simulink model "DTC"  (R2023a)
settings: Solver=FixedStepAuto  StartTime=0.0  StopTime=6  FixedStep=Ts  MaxStep=1e-4  RelTol=1e-3
PreLoadFcn:
  | Ts=1e-5;
InitFcn:
  | Ts=1e-5;
undefined symbols (not defined in the file): DiscIntNeverNeededParam
libraries: spsIGBTDiodeLib x6, slpidlib x2, spsAsynchronousMachineSIUnitsLib x1, simulink x1, spsDCVoltageSourceLib x1, spsVoltageMeasurementLib x1, sps_lib x1
Description:
  | Copyright 2011-2013 Ruan Jiayang, Tsinghua Univ.
settings Model: ExtModeTrigMode=oneshot  Creator=Hoang Lehuy, Laval University  LastModifiedBy=搬砖工卢卡斯
settings SolverCC: AlgebraicLoopSolver=TrustRegion
settings DataIOCC: SaveFinalState=on  SaveFormat=Array  SignalLoggingSaveFormat=ModelDataLogs  SaveOutput=off  SaveTime=off  ReturnWorkspaceOutputs=off  SignalLoggingName=sigsOut
settings OptimizationCC: BlockReduction=off  ExpressionDepthLimit=2147483647  InitFltsAndDblsToZero=on  LifeSpan=inf
settings DebuggingCC: SaveWithParameterizedLinksMsg=none  UnderspecifiedInitializationDetection=Classic  MergeDetectMultiDrivingBlocksExec=none  CheckExecutionContextPreStartOutputMsg=on  SignalResolutionControl=TryResolveAllWithWarning  MultiTaskDSMMsg=warning  MultiTaskCondExecSysMsg=none  FcnCallInpInsideContextMsg=warning  UnconnectedInputMsg=warning  UnconnectedLineMsg=warning  StateNameClashWarn=warning  SFUnexpectedBacktrackingDiag=warning  SFNoUnconditionalDefaultTransitionDiag=warning  SFExecutionAtInitializationDiag=none  ArithmeticOperatorsInVariantConditions=warning
settings HardwareCC: ProdBitPerPointer=32  ProdBitPerSizeT=32  ProdBitPerPtrDiffT=32  ProdLargestAtomicFloat=None  ProdIntDivRoundTo=Undefined  ProdEndianess=Unspecified  ProdWordSize=32  ProdHWDeviceType=32-bit Generic  TargetUnknown=on
settings ModelReferenceCC: PropagateSignalLabelsOutOfModel=off
settings SFSimCC: SimUseLocalCustomCode=off  SimParseCustomCode=off  CustomCodeUndefinedFunction=UseInterfaceOnly
settings RTWCC: RTWUseLocalCustomCode=off
settings CodeAppCC: StateflowObjectComments=on
settings GRTTargetCC: TargetFcnLib=ansi_tfl_tmw.mat  TargetLangStandard=C89/C90 (ANSI)  CombineOutputUpdateFcns=off  GRTInterface=on
settings ConfigComp: CovMetricSettings=dw  CovSaveCumulativeToWorkspaceVar=on  CovSaveSingleToWorkspaceVar=on  CovExternalEMLEnable=off

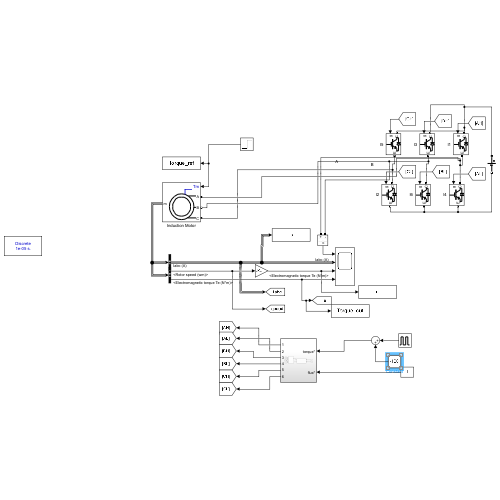
[thumbnail: Simulink's stored preview of the top-level diagram]
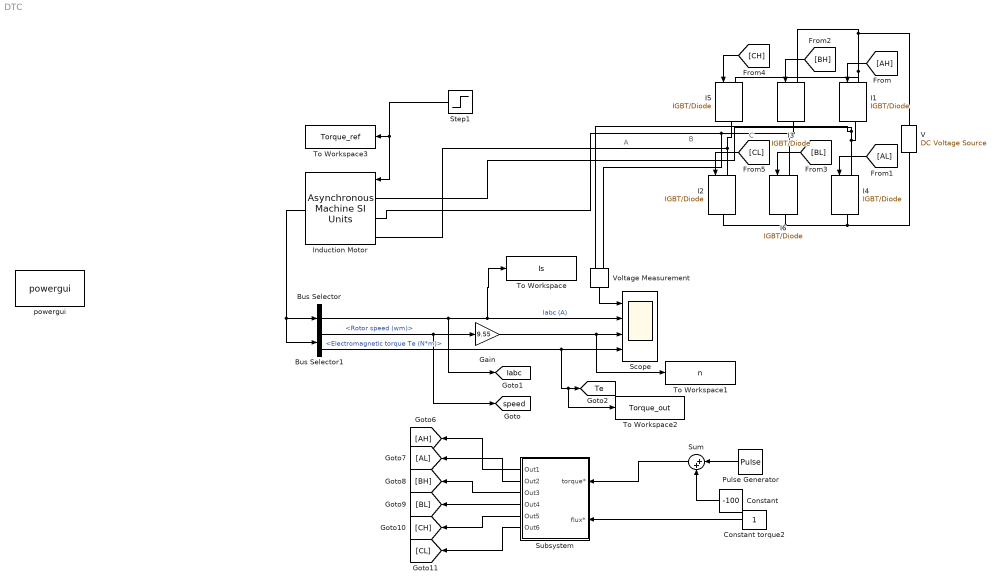
== system DTC ==
  note: B
  note: A
  note: C
  Bus Selector : BusSelector  OutputSignals=Stator measurements.Stator current is_a (A),Stator measurements.Stator current is_b (A),Stator measurements.Stator current is_c (A)  OutputAsBus=on
  Bus Selector1 : BusSelector  OutputSignals=Mechanical.Rotor speed (wm),Mechanical.Electromagnetic torque Te (N*m)
  Constant : Constant  Value=-100
  Constant torque2 : Constant
  Gain : Gain  Gain=9.55
  I{1..6} (6 alike) : spsIGBTDiodeLib/IGBT//Diode  Ron=1e-3  Rs=1e5  Cs=inf  Measurements=off
  "Induction Motor " : spsAsynchronousMachineSIUnitsLib/Asynchronous Machine SI Units  RotorType=Squirrel-cage  PresetModel=No  MechanicalLoad=Torque Tm  ShowDetailedParameters=on  ReferenceFrame=Stationary  Units=SI  MeasurementBus=off  NominalParameters=[ 2000, 346, 60 ]  VoltageRatio=1  Stator=[ 0.087 0.8e-3 ]  Rotor="[ 0.228  0.8e-3 ]"  Cage1=[0.4155 0.002066]  Cage2=[0.4168 0.0003495]  Lm=34.7e-3  Mechanical="[1.662  0.01 2 ]"  PolePairs=2  InitialConditions="[ 1, 0 ,  0 , 0 , 0 , 0 , 0 , 0 ]"  SimulateSaturation=off  Saturation=[0 0;0 0]  LoadFlowParameters=0  TsPowergui=0  TsBlock=-1  IterativeModel=Trapezoidal non iterative  IterativeDiscreteModel=Trapezoidal non iterative  Pmec=1.492e+006
      settings: AttributesFormatString=\n
  Pulse Generator : DiscretePulseGenerator  PulseType=Time based  Amplitude=200  PulseWidth=50
  Scope : Scope  NumInputPorts=4
  Step1 : Step  Time=1.5  After=0  SampleTime=0
  Subsystem : Subsystem
  Sum : Sum  Inputs=|++
  To Workspace : ToWorkspace  VariableName=Is  SaveFormat=Timeseries  SampleTime=-1
  To Workspace1 : ToWorkspace  VariableName=n  SaveFormat=Timeseries  SampleTime=-1
  To Workspace2 : ToWorkspace  VariableName=Torque_out  SaveFormat=Timeseries  SampleTime=-1
  To Workspace3 : ToWorkspace  VariableName=Torque_ref  SaveFormat=Timeseries  SampleTime=-1
  V : spsDCVoltageSourceLib/DC Voltage Source  Amplitude=530  Measurements=None
  Voltage Measurement : spsVoltageMeasurementLib/Voltage Measurement  PhasorSimulation=off  OutputType=Complex  PSBequivalent=0
  powergui : sps_lib/powergui  Priority=2  SimulationMode=Discrete  SampleTime=Ts  frequency=60  Iterations=50  frequencyindice=0  Pbase=100e6  ErrMax=1e-4  UnitsV=kV  UnitsW=MW  buscounter=0  FunctionMessages=off  echomessages=off  EnableUseOfTLC=off  CurrentSourceSwitches=on  DisableSnubberDevices=off  DisableRonSwitches=off  DisableVfSwitches=off  DisplayEquations=off  AutomaticDiscreteSolvers=off  SolverType=Tustin/Backward Euler (TBE)  Interpol=off  ExternalGateDelay=off  methode=off  Ts=0  x0status=blocks  SPID=off  SwTol=0  HookPort=off  NonlinearTolerance=1e-4  nMaxIteration=100  ContinueOnMaxIteration=off  RestoreLinks=warning  ResistiveCurrentMeasurement=off  Frange=[0:2:500]  Ylog=off  Xlog=on  ShowGrid=off  save=off  variable=ZData  structure=0  ZoomFFT=on  StartTime=0.0  cycles=1  DisplayStyle=off  fundamental=60  FreqAxis=off  MaxFrequency=1000  frequencyindicesteady=1  RmsSteady=1  display=off
  tag scope: Iabc=global, Te=global, speed=global
  wires:
  Bus Selector1/1 -> Gain/1, [speed]  "<Rotor speed (wm)>"
  Bus Selector/1 -> [Iabc], To Workspace/1, Scope/2  "Iabc (A)"
  Bus Selector1/2 -> Scope/4, To Workspace2/1, [Te]  "<Electromagnetic torque Te (N*m)>"
  "Induction Motor "/1 -> Bus Selector1/1, Bus Selector/1
  Gain/1 -> To Workspace1/1, Scope/3
  Constant torque2/1 -> Subsystem/2(flux*)
  Step1/1 -> "Induction Motor "/1, To Workspace3/1
  Voltage Measurement/1 -> Scope/1
  [CH] -> I5/1
  [BL] -> I6/1
  [BH] -> I3/1
  [AL] -> I4/1
  [CL] -> I2/1
  [AH] -> I1/1
  Subsystem/1(Out1) -> [AH]
  Subsystem/2(Out2) -> [AL]
  Subsystem/3(Out3) -> [BH]
  Subsystem/4(Out4) -> [BL]
  Subsystem/5(Out5) -> [CH]
  Subsystem/6(Out6) -> [CL]
  Pulse Generator/1 -> Sum/1
  Constant/1 -> Sum/2
  Sum/1 -> Subsystem/1(torque*)
  connections:
  Voltage Measurement/LConn2 -- I6/LConn1 -- I3/RConn1 -- "Induction Motor "/LConn2
  I3/LConn1 -- V/RConn1 -- I5/LConn1 -- I1/LConn1
  I4/RConn1 -- V/LConn1 -- I2/RConn1 -- I6/RConn1
  Voltage Measurement/LConn1 -- "Induction Motor "/LConn1 -- I1/RConn1 -- I4/LConn1
  I5/RConn1 -- "Induction Motor "/LConn3 -- I2/LConn1

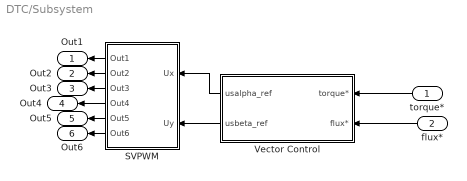
== system DTC/Subsystem ==
  torque* : Inport
  flux* : Inport  Port=2
  SVPWM : Subsystem
  Vector Control : Subsystem
  Out1 : Outport
  Out2 : Outport  Port=2
  Out3 : Outport  Port=3
  Out4 : Outport  Port=4
  Out5 : Outport  Port=5
  Out6 : Outport  Port=6
  wires:
  SVPWM/1(Out1) -> Out1/1
  SVPWM/5(Out5) -> Out5/1
  SVPWM/6(Out6) -> Out6/1
  flux*/1 -> Vector Control/2(flux*)
  Vector Control/2(usbeta_ref) -> SVPWM/2(Uy)
  Vector Control/1(usalpha_ref) -> SVPWM/1(Ux)
  torque*/1 -> Vector Control/1(torque*)
  SVPWM/2(Out2) -> Out2/1
  SVPWM/4(Out4) -> Out4/1
  SVPWM/3(Out3) -> Out3/1

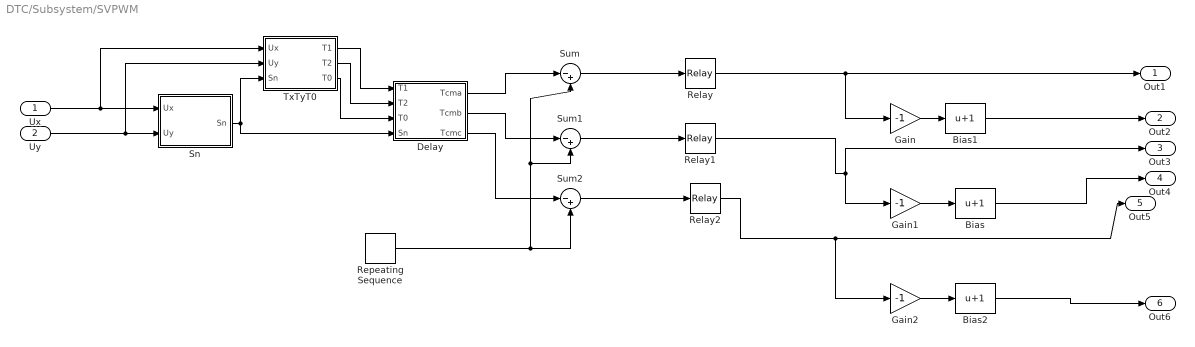
== system DTC/Subsystem/SVPWM ==
  Ux : Inport
  Uy : Inport  Port=2
  Bias : Bias  Bias=1  SaturateOnIntegerOverflow=off
  Bias1 : Bias  Bias=1  SaturateOnIntegerOverflow=off
  Bias2 : Bias  Bias=1  SaturateOnIntegerOverflow=off
  Delay : MATLAB Function  TreatAsAtomicUnit=on
  Gain : Gain  Gain=-1
  Gain1 : Gain  Gain=-1
  Gain2 : Gain  Gain=-1
  Relay : Relay  OnSwitchValue=0  OffSwitchValue=0
  Relay1 : Relay  OnSwitchValue=0  OffSwitchValue=0
  Relay2 : Relay  OnSwitchValue=0  OffSwitchValue=0
  Repeating Sequence : simulink/Sources/Repeating Sequence  rep_seq_t=[0 1/2000/2 1/2000]  rep_seq_y=[0 1/2000/2 0]
  Sn : MATLAB Function  TreatAsAtomicUnit=on
  Sum : Sum  Inputs=|-+
  Sum1 : Sum  Inputs=|-+
  Sum2 : Sum  Inputs=|-+
  TxTyT0 : MATLAB Function  TreatAsAtomicUnit=on
  Out1 : Outport
  Out2 : Outport  Port=2
  Out3 : Outport  Port=3
  Out4 : Outport  Port=4
  Out5 : Outport  Port=5
  Out6 : Outport  Port=6
  wires:
  Delay/1(Tcma) -> Sum/1
  Delay/2(Tcmb) -> Sum1/1
  Delay/3(Tcmc) -> Sum2/1
  Repeating Sequence/1 -> Sum/2, Sum1/2, Sum2/2
  Sum/1 -> Relay/1
  Sum2/1 -> Relay2/1
  Sum1/1 -> Relay1/1
  Relay1/1 -> Out3/1, Gain1/1
  Relay2/1 -> Out5/1, Gain2/1
  Sn/1(Sn) -> TxTyT0/3(Sn), Delay/4(Sn)
  TxTyT0/1(T1) -> Delay/1(T1)
  TxTyT0/2(T2) -> Delay/2(T2)
  TxTyT0/3(T0) -> Delay/3(T0)
  Gain1/1 -> Bias/1
  Gain/1 -> Bias1/1
  Gain2/1 -> Bias2/1
  Bias1/1 -> Out2/1
  Bias/1 -> Out4/1
  Bias2/1 -> Out6/1
  Relay/1 -> Out1/1, Gain/1
  Ux/1 -> Sn/1(Ux), TxTyT0/1(Ux)
  Uy/1 -> Sn/2(Uy), TxTyT0/2(Uy)

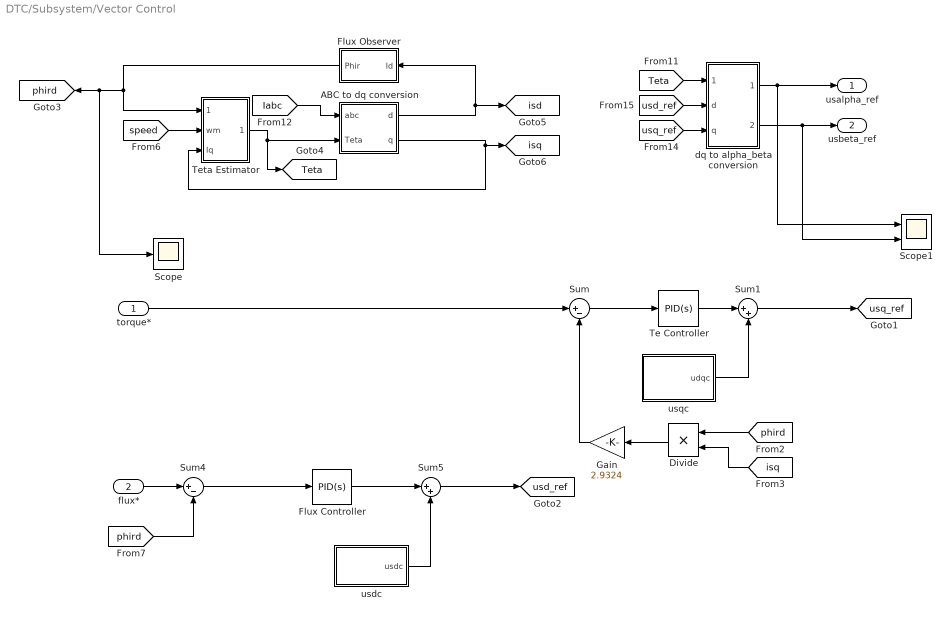
== system DTC/Subsystem/Vector Control ==
  torque* : Inport
  flux* : Inport  Port=2
  ABC to dq conversion : Subsystem
  Divide : Product
  Flux Controller : slpidlib/PID Controller  Controller=PID  Form=Parallel  TimeDomain=Continuous-time  UseExternalTs=off  SampleTime=1  IntegratorMethod=Forward Euler  FilterMethod=Forward Euler  ControllerParametersSource=internal  P=138.2107  I=247.3835  UseKiTs=off  D=0  N=100  UseFilter=on  TunerSelectOption=Transfer Function Based (PID Tuner App)  InitialConditionSource=internal  InitialConditionForIntegrator=100  InitialConditionForFilter=0  DifferentiatorICPrevScaledInput=0  ExternalReset=none  TrackingMode=off  Kt=1  LimitOutput=on  SatLimitsSource=internal  UpperSaturationLimit=200  LowerSaturationLimit=-200  LinearizeAsGain=off  AntiWindupMode=clamping  Kb=1  LimitIntegrator=off  UpperIntegratorSaturationLimit=inf  LowerIntegratorSaturationLimit=-inf  POutMin=[]  POutMax=[]  IOutMin=[]  IOutMax=[]  DOutMin=[]  DOutMax=[]  NOutMin=[]  NOutMax=[]  SumOutMin=[]  SumOutMax=[]  SaturationOutMin=[]  SaturationOutMax=[]  PParamMin=[]  PParamMax=[]  IParamMin=[]  IParamMax=[]  DParamMin=[]  DParamMax=[]  NParamMin=[]  NParamMax=[]  KbParamMin=[]  KbParamMax=[]  KtParamMin=[]  KtParamMax=[]  KbOutMin=[]  KbOutMax=[]  KtOutMin=[]  KtOutMax=[]  IntegratorOutMin=[]  IntegratorOutMax=[]  FilterOutMin=[]  FilterOutMax=[]  SumI1OutMin=[]  SumI1OutMax=[]  SumI2OutMin=[]  SumI2OutMax=[]  SumI3OutMin=[]  SumI3OutMax=[]  SumI4OutMin=[]  SumI4OutMax=[]  SumDOutMin=[]  SumDOutMax=[]  DifferentiatorOutMin=[]  DifferentiatorOutMax=[]  FilterDiffOutCoefMin=[]  FilterDiffOutCoefMax=[]  ReciprocalOutMin=[]  ReciprocalOutMax=[]  SumDenOutMin=[]  SumDenOutMax=[]  SumNumOutMin=[]  SumNumOutMax=[]  DivideOutMin=[]  DivideOutMax=[]  UdiffTsProdOutMin=[]  UdiffTsProdOutMax=[]  NTsProdOutMin=[]  NTsProdOutMax=[]  UintegralTsProdOutMin=[]  UintegralTsProdOutMax=[]  UngainTsProdOutMin=[]  UngainTsProdOutMax=[]  ClampingZeroOutDataTypeStr=Inherit: Inherit via back propagation  ClampingZeroOutMin=[]  ClampingZeroOutMax=[]  FilterDenConstantOutDataTypeStr=Inherit: Inherit via back propagation  FilterDenConstantOutMin=[]  FilterDenConstantOutMax=[]  PCopyOutDataTypeStr=Inherit: Inherit via back propagation  PCopyOutMin=[]  PCopyOutMax=[]  NCopyOutDataTypeStr=Inherit: Inherit via back propagation  NCopyOutMin=[]  NCopyOutMax=[]  IntegratorContinuousStateAttributes=''  IntegratorStateMustResolveToSignalObject=off  IntegratorRTWStateStorageClass=Auto  FilterContinuousStateAttributes=''  FilterStateMustResolveToSignalObject=off  FilterRTWStateStorageClass=Auto  ParallelPVariant=InternalParameters  IdealPVariant=Disabled  IVariant=InternalParameters  DVariant=InternalParameters  IntegratorVariant=Continuous  SatVariant=Enabled  AWVariant=ContClampingParallel  PCopyVariant=Disabled  TRVariant=Disabled  FdbkBlocksVariant=Forward  IdealPFdbkVariant=Disabled  SatFdbkVariant=Disabled  DerivativeFilterVariant=ContFilter  NVariant=InternalParameters  NCopyVariant=Disabled  FilterICVariant=InternalICsFilter  IntegratorICVariant=InternalICs  ExternalResetVariant=Disabled  TRSumVariant=Passthrough  SumFdbkVariant=Disabled  SumVariant=Sum_PID  TsampFilterVariant=InternalTs  TsampNgainVariant=Passthrough  TsampIntegralVariant=Disabled_SignalSpec  ExternalSaturationOutDataTypeStr=Inherit: Same as second input
  Flux Observer : Subsystem  mask(Flux Calcultation){}
      mask init:
      | NF=0.44572610323020e-6;
      | DF=[1 -0.99998715486734];
  Gain : Gain  Gain=2.9324
  Scope : Scope
  Scope1 : Scope  NumInputPorts=2
  Sum : Sum  Inputs=|+-
  Sum1 : Sum  Inputs=|++
  Sum4 : Sum  Inputs=|+-
  Sum5 : Sum  Inputs=|++
  Te Controller : slpidlib/PID Controller  Controller=PID  Form=Parallel  TimeDomain=Continuous-time  UseExternalTs=off  SampleTime=1  IntegratorMethod=Forward Euler  FilterMethod=Forward Euler  ControllerParametersSource=internal  P=2.69732  I=148.34534  UseKiTs=off  D=0  N=100  UseFilter=on  TunerSelectOption=Transfer Function Based (PID Tuner App)  InitialConditionSource=internal  InitialConditionForIntegrator=100  InitialConditionForFilter=0  DifferentiatorICPrevScaledInput=0  ExternalReset=none  TrackingMode=off  Kt=1  LimitOutput=on  SatLimitsSource=internal  UpperSaturationLimit=200  LowerSaturationLimit=-200  LinearizeAsGain=off  AntiWindupMode=clamping  Kb=1  LimitIntegrator=off  UpperIntegratorSaturationLimit=inf  LowerIntegratorSaturationLimit=-inf  POutMin=[]  POutMax=[]  IOutMin=[]  IOutMax=[]  DOutMin=[]  DOutMax=[]  NOutMin=[]  NOutMax=[]  SumOutMin=[]  SumOutMax=[]  SaturationOutMin=[]  SaturationOutMax=[]  PParamMin=[]  PParamMax=[]  IParamMin=[]  IParamMax=[]  DParamMin=[]  DParamMax=[]  NParamMin=[]  NParamMax=[]  KbParamMin=[]  KbParamMax=[]  KtParamMin=[]  KtParamMax=[]  KbOutMin=[]  KbOutMax=[]  KtOutMin=[]  KtOutMax=[]  IntegratorOutMin=[]  IntegratorOutMax=[]  FilterOutMin=[]  FilterOutMax=[]  SumI1OutMin=[]  SumI1OutMax=[]  SumI2OutMin=[]  SumI2OutMax=[]  SumI3OutMin=[]  SumI3OutMax=[]  SumI4OutMin=[]  SumI4OutMax=[]  SumDOutMin=[]  SumDOutMax=[]  DifferentiatorOutMin=[]  DifferentiatorOutMax=[]  FilterDiffOutCoefMin=[]  FilterDiffOutCoefMax=[]  ReciprocalOutMin=[]  ReciprocalOutMax=[]  SumDenOutMin=[]  SumDenOutMax=[]  SumNumOutMin=[]  SumNumOutMax=[]  DivideOutMin=[]  DivideOutMax=[]  UdiffTsProdOutMin=[]  UdiffTsProdOutMax=[]  NTsProdOutMin=[]  NTsProdOutMax=[]  UintegralTsProdOutMin=[]  UintegralTsProdOutMax=[]  UngainTsProdOutMin=[]  UngainTsProdOutMax=[]  ClampingZeroOutDataTypeStr=Inherit: Inherit via back propagation  ClampingZeroOutMin=[]  ClampingZeroOutMax=[]  FilterDenConstantOutDataTypeStr=Inherit: Inherit via back propagation  FilterDenConstantOutMin=[]  FilterDenConstantOutMax=[]  PCopyOutDataTypeStr=Inherit: Inherit via back propagation  PCopyOutMin=[]  PCopyOutMax=[]  NCopyOutDataTypeStr=Inherit: Inherit via back propagation  NCopyOutMin=[]  NCopyOutMax=[]  IntegratorContinuousStateAttributes=''  IntegratorStateMustResolveToSignalObject=off  IntegratorRTWStateStorageClass=Auto  FilterContinuousStateAttributes=''  FilterStateMustResolveToSignalObject=off  FilterRTWStateStorageClass=Auto  ParallelPVariant=InternalParameters  IdealPVariant=Disabled  IVariant=InternalParameters  DVariant=InternalParameters  IntegratorVariant=Continuous  SatVariant=Enabled  AWVariant=ContClampingParallel  PCopyVariant=Disabled  TRVariant=Disabled  FdbkBlocksVariant=Forward  IdealPFdbkVariant=Disabled  SatFdbkVariant=Disabled  DerivativeFilterVariant=ContFilter  NVariant=InternalParameters  NCopyVariant=Disabled  FilterICVariant=InternalICsFilter  IntegratorICVariant=InternalICs  ExternalResetVariant=Disabled  TRSumVariant=Passthrough  SumFdbkVariant=Disabled  SumVariant=Sum_PID  TsampFilterVariant=InternalTs  TsampNgainVariant=Passthrough  TsampIntegralVariant=Disabled_SignalSpec  ExternalSaturationOutDataTypeStr=Inherit: Same as second input
  Teta Estimator : Subsystem
  dq to alpha_beta conversion : Subsystem
  usdc : Subsystem
  usqc : Subsystem
  usalpha_ref : Outport
  usbeta_ref : Outport  Port=2
  tag scope: Teta=global, isd=global, isq=global, phird=global, usd_ref=global, usq_ref=global
  wires:
  Sum/1 -> Te Controller/1
  Te Controller/1 -> Sum1/1
  usqc/1(udqc) -> Sum1/2
  Gain/1 -> Sum/2
  Sum1/1 -> [usq_ref]
  flux*/1 -> Sum4/1
  [phird] -> Sum4/2
  Sum4/1 -> Flux Controller/1
  Flux Controller/1 -> Sum5/1
  Sum5/1 -> [usd_ref]
  Flux Observer/1(Phir) -> Teta Estimator/1(Phird), [phird], Scope/1
  Teta Estimator/1(Teta) -> ABC to dq conversion/2(Teta), [Teta]
  [speed] -> Teta Estimator/2(wm)
  [Iabc] -> ABC to dq conversion/1(abc)
  [Teta] -> dq to alpha_beta conversion/1(Teta)
  ABC to dq conversion/2(q) -> Teta Estimator/3(Iq), [isq]
  [usd_ref] -> dq to alpha_beta conversion/2(d)
  [usq_ref] -> dq to alpha_beta conversion/3(q)
  usdc/1(usdc) -> Sum5/2
  dq to alpha_beta conversion/1(usalpha) -> usalpha_ref/1, Scope1/1
  dq to alpha_beta conversion/2(usbeta) -> usbeta_ref/1, Scope1/2
  Divide/1 -> Gain/1
  [phird] -> Divide/1
  [isq] -> Divide/2
  ABC to dq conversion/1(d) -> [isd], Flux Observer/1(Id)
  torque*/1 -> Sum/1

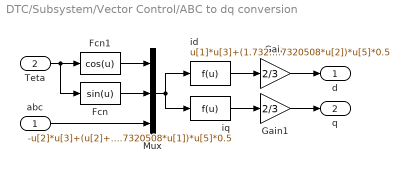
== system DTC/Subsystem/Vector Control/ABC to dq conversion ==
  abc : Inport
  Teta : Inport  Port=2
  Fcn : Fcn  Expr=sin(u)
  Fcn1 : Fcn  Expr=cos(u)
  Gain : Gain  Gain=2/3  SaturateOnIntegerOverflow=on  OutDataTypeStr=Inherit: Same as input  ParamDataTypeStr=Inherit: Same as input
  Gain1 : Gain  Gain=2/3  SaturateOnIntegerOverflow=on  OutDataTypeStr=Inherit: Same as input  ParamDataTypeStr=Inherit: Same as input
  Mux : Mux  Inputs=[1 1 3]
  id : Fcn  Expr=u[1]*u[3]+(1.7320508*u[2]-u[1])*u[4]*0.5+(-u[1]-1.7320508*u[2])*u[5]*0.5
  iq : Fcn  Expr=-u[2]*u[3]+(u[2]+1.7320508*u[1])*u[4]*0.5+(u[2]-1.7320508*u[1])*u[5]*0.5
  d : Outport  InitialOutput=0
  q : Outport  Port=2  InitialOutput=0
  wires:
  Fcn/1 -> Mux/2
  Fcn1/1 -> Mux/1
  Teta/1 -> Fcn1/1, Fcn/1
  Mux/1 -> iq/1, id/1
  abc/1 -> Mux/3
  iq/1 -> Gain1/1
  id/1 -> Gain/1
  Gain/1 -> d/1
  Gain1/1 -> q/1

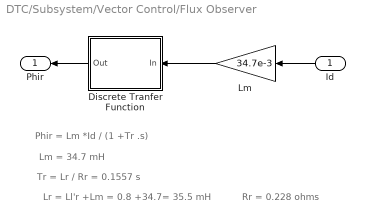
== system DTC/Subsystem/Vector Control/Flux Observer ==
  note: Phir = Lm *Id / (1 +Tr .s)
  note: Lm = 34.7 mH
  note: Lr = Ll'r +Lm = 0.8 +34.7= 35.5 mH
  note: Tr = Lr / Rr = 0.1557 s
  note: Rr = 0.228 ohms
  Id : Inport
  Discrete Tranfer Function : Subsystem  mask(First Order Low Pass Filter (Discrete)){T=0.1557, Ts=Ts}
      mask prompts: T "Time constant T (s) :"; Ts "Time step (s)"
      mask help: H(s)=1/(1+T.s)
      mask init:
      | X=[0 1 2 3 4];
      |  Y=[-2 -2 -3 -4 -4];
      |  str=sprintf('\nH=1/(1+T.s)\n T= %g s\n\n\n',T);
      | num=1;
      | den=[T 1];
      | 
      | % discrete transfer function
      | % descending powers of z
      | numd= Ts/T;
      | dend=[ 1  (Ts-T)/T];
      mask Display:
      | plot(X,Y);
      | disp(str);
  Lm : Gain  Gain=34.7e-3  SaturateOnIntegerOverflow=on  OutDataTypeStr=Inherit: Same as input  ParamDataTypeStr=Inherit: Same as input
  Phir : Outport
  wires:
  Discrete Tranfer Function/1(Out) -> Phir/1
  Id/1 -> Lm/1
  Lm/1 -> Discrete Tranfer Function/1(In)

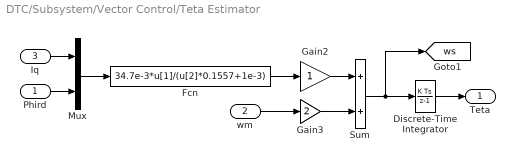
== system DTC/Subsystem/Vector Control/Teta Estimator ==
  Phird : Inport
  wm : Inport  Port=2
  Iq : Inport  Port=3
  Discrete-Time Integrator : DiscreteIntegrator  SampleTime=Ts  ICPrevOutput=DiscIntNeverNeededParam  ICPrevScaledInput=DiscIntNeverNeededParam
  Fcn : Fcn  Expr=34.7e-3*u[1]/(u[2]*0.1557+1e-3)
  Gain2 : Gain  SaturateOnIntegerOverflow=on  OutDataTypeStr=Inherit: Same as input  ParamDataTypeStr=Inherit: Same as input
  Gain3 : Gain  Gain=2  SaturateOnIntegerOverflow=on  OutDataTypeStr=Inherit: Same as input  ParamDataTypeStr=Inherit: Same as input
  Mux : Mux  Inputs=2
  Sum : Sum  InputSameDT=on  SaturateOnIntegerOverflow=on  OutDataTypeStr=Inherit: Same as first input
  Teta : Outport  InitialOutput=0
  tag scope: ws=global
  wires:
  Discrete-Time Integrator/1 -> Teta/1
  Sum/1 -> Discrete-Time Integrator/1, [ws]
  Gain3/1 -> Sum/2
  Gain2/1 -> Sum/1
  wm/1 -> Gain3/1
  Fcn/1 -> Gain2/1
  Phird/1 -> Mux/2
  Iq/1 -> Mux/1
  Mux/1 -> Fcn/1

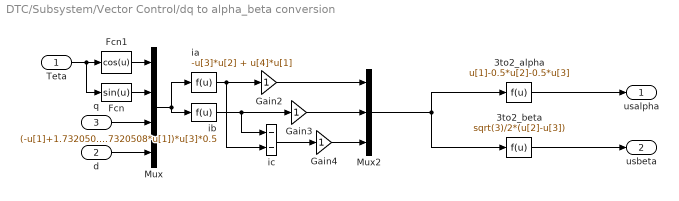
== system DTC/Subsystem/Vector Control/dq to alpha_beta conversion ==
  Teta : Inport
  d : Inport  Port=2
  q : Inport  Port=3
  3to2_alpha : Fcn  Expr=u[1]-0.5*u[2]-0.5*u[3]
  3to2_beta : Fcn  Expr=sqrt(3)/2*(u[2]-u[3])
  Fcn : Fcn  Expr=sin(u)
  Fcn1 : Fcn  Expr=cos(u)
  Gain2 : Gain  SaturateOnIntegerOverflow=on  OutDataTypeStr=Inherit: Same as input  ParamDataTypeStr=Inherit: Same as input
  Gain3 : Gain  SaturateOnIntegerOverflow=on  OutDataTypeStr=Inherit: Same as input  ParamDataTypeStr=Inherit: Same as input
  Gain4 : Gain  SaturateOnIntegerOverflow=on  OutDataTypeStr=Inherit: Same as input  ParamDataTypeStr=Inherit: Same as input
  Mux : Mux
  Mux2 : Mux  Inputs=3
  ia : Fcn  Expr=-u[3]*u[2] + u[4]*u[1]
  ib : Fcn  Expr=(-u[1]+1.7320508*u[2])*u[4]*0.5+(u[2]+1.7320508*u[1])*u[3]*0.5
  ic : Sum  Inputs=--  InputSameDT=on  SaturateOnIntegerOverflow=on  OutDataTypeStr=Inherit: Same as first input
  usalpha : Outport
  usbeta : Outport  Port=2
  wires:
  Fcn/1 -> Mux/2
  Fcn1/1 -> Mux/1
  Mux/1 -> ib/1, ia/1
  Teta/1 -> Fcn1/1, Fcn/1
  q/1 -> Mux/3
  d/1 -> Mux/4
  Gain3/1 -> Mux2/2
  ic/1 -> Gain4/1
  Gain4/1 -> Mux2/3
  Gain2/1 -> Mux2/1
  ia/1 -> Gain2/1, ic/2
  ib/1 -> Gain3/1, ic/1
  Mux2/1 -> 3to2_alpha/1, 3to2_beta/1
  3to2_alpha/1 -> usalpha/1
  3to2_beta/1 -> usbeta/1

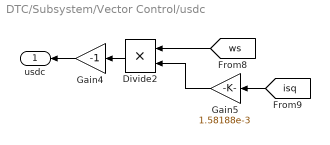
== system DTC/Subsystem/Vector Control/usdc ==
  Divide2 : Product
  Gain4 : Gain  Gain=-1
  Gain5 : Gain  Gain=1.58188e-3
  usdc : Outport
  wires:
  Divide2/1 -> Gain4/1
  [ws] -> Divide2/1
  [isq] -> Gain5/1
  Gain5/1 -> Divide2/2
  Gain4/1 -> usdc/1

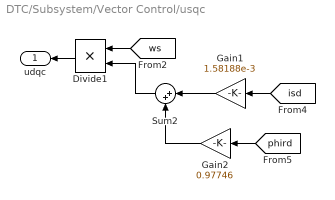
== system DTC/Subsystem/Vector Control/usqc ==
  Divide1 : Product
  Gain1 : Gain  Gain=1.58188e-3
  Gain2 : Gain  Gain=0.97746
  Sum2 : Sum  Inputs=|++
  udqc : Outport
  wires:
  [ws] -> Divide1/1
  Sum2/1 -> Divide1/2
  Gain1/1 -> Sum2/1
  Gain2/1 -> Sum2/2
  [isd] -> Gain1/1
  [phird] -> Gain2/1
  Divide1/1 -> udqc/1

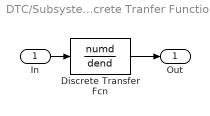
== system DTC/Subsystem/Vector Control/Flux Observer/Discrete Tranfer Function ==
  In : Inport
  Discrete Transfer Fcn : DiscreteTransferFcn  Numerator=numd  Denominator=dend  SampleTime=Ts
  Out : Outport  InitialOutput=0
  wires:
  Discrete Transfer Fcn/1 -> Out/1
  In/1 -> Discrete Transfer Fcn/1

== matlab function DTC/Subsystem/SVPWM/Sn ==
  data: Sn output; Ux input; Uy input
function Sn = S(Ux,Uy)
theta=atan2(Uy,Ux)*180/pi;
if theta>=0&&theta<60
    Sn=1;
elseif theta>=60&&theta<120
    Sn=2;
elseif theta>=120&&theta<180
    Sn=3;
elseif theta>=-180&&theta<-120
    Sn=4;
elseif theta>=-120&&theta<-60
    Sn=5;
else Sn=6;
end

== matlab function DTC/Subsystem/SVPWM/TxTyT0 ==
  data: Ux input; Uy input; Sn input; T1 output; T2 output; T0 output
function [T1,T2,T0]=T(Ux,Uy,Sn)
Ts=1/2000;
Udc=530;

X=sqrt(3)*Ts/Udc*Uy;
Y=sqrt(3)*Ts/2/Udc*(sqrt(3)*Ux+Uy);
Z=sqrt(3)*Ts/2/Udc*(-sqrt(3)*Ux+Uy);

if Sn==1
    T1=-Z;T2=X;
elseif Sn==2;
    T1=Z;T2=Y;
elseif Sn==3;
    T1=X;T2=-Y;
elseif Sn==4;
    T1=-X;T2=Z;
elseif Sn==5;
    T1=-Y;T2=-Z;
else T1=Y;T2=-X;
end
    
if T1+T2>Ts
    a=T1;b=T2;
    T1=a*Ts/(a+b);
    T2=b*Ts/(a+b);
end

T0=Ts-T1-T2;

== matlab function DTC/Subsystem/SVPWM/Delay ==
  data: T1 input; T2 input; T0 input; Tcma output; Tcmb output; Tcmc output; Sn input
function [Tcma,Tcmb,Tcmc]=D(T1,T2,T0,Sn)
T=1/2000;
Udc=530;
ton1=0.25*T0;
ton2=ton1+T1/2;
ton3=ton2+T2/2;
if Sn==1
    Tcma=ton1;Tcmb=ton2;Tcmc=ton3;
elseif Sn==2;
    Tcma=ton2;Tcmb=ton1;Tcmc=ton3;
elseif Sn==3;
    Tcma=ton3;Tcmb=ton1;Tcmc=ton2;
elseif Sn==4;
    Tcma=ton3;Tcmb=ton2;Tcmc=ton1;
elseif Sn==5;
    Tcma=ton2;Tcmb=ton3;Tcmc=ton1;
else Tcma=ton1;Tcmb=ton3;Tcmc=ton2;
end
